simulink model "AeroModel"  (R2024b)
settings: Solver=VariableStepAuto  StartTime=0.0  StopTime=10.0  RelTol=1e-3
settings Model: Creator=ewise  LastModifiedBy=ewise

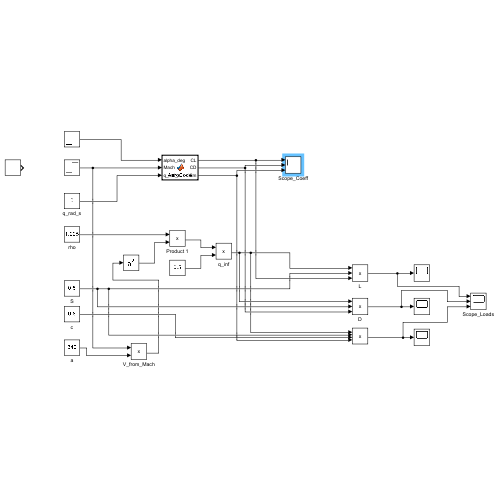
[thumbnail: Simulink's stored preview of the top-level diagram]
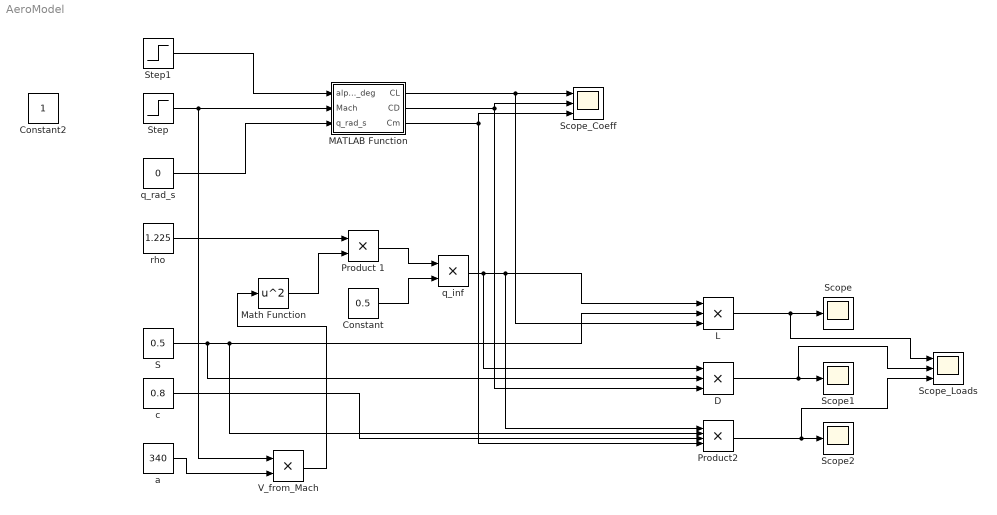
== system AeroModel ==
  Constant : Constant  Value=0.5
  Constant2 : Constant
  D : Product  Inputs=3
  L : Product  Inputs=3
  MATLAB Function : MATLAB Function  TreatAsAtomicUnit=on
  Math Function : Math  Operator=square
  Product 1 : Product
  Product2 : Product  Inputs=4
  S : Constant  Value=0.5
  Scope : Scope
  Scope1 : Scope
  Scope2 : Scope
  Scope_Coeff : Scope  NumInputPorts=3
  Scope_Loads : Scope  NumInputPorts=3
  Step : Step  Time=3  Before=4  After=7  SampleTime=0
  Step1 : Step  Time=2  Before=2  After=12  SampleTime=0
  V_from_Mach : Product
  a : Constant  Value=340
  c : Constant  Value=0.8
  q_inf : Product
  q_rad_s : Constant  Value=0
  rho : Constant  Value=1.225
  wires:
  Step/1 -> V_from_Mach/1, MATLAB Function/2(Mach)
  q_rad_s/1 -> MATLAB Function/3(q_rad_s)
  MATLAB Function/2(CD) -> Scope_Coeff/2, D/3
  MATLAB Function/3(Cm) -> Product2/4, Scope_Coeff/3
  rho/1 -> Product 1/1
  Math Function/1 -> Product 1/2
  Product 1/1 -> q_inf/1
  Constant/1 -> q_inf/2
  q_inf/1 -> D/1, Product2/1, L/1
  S/1 -> D/2, Product2/2, L/2
  MATLAB Function/1(CL) -> Scope_Coeff/1, L/3
  c/1 -> Product2/3
  L/1 -> Scope_Loads/1, Scope/1
  D/1 -> Scope_Loads/2, Scope1/1
  Product2/1 -> Scope_Loads/3, Scope2/1
  a/1 -> V_from_Mach/2
  V_from_Mach/1 -> Math Function/1
  Step1/1 -> MATLAB Function/1(alpha_deg)

== matlab function AeroModel/MATLAB Function ==
  data: alpha_deg input; CL output; Mach input; q_rad_s input; CD output; Cm output
function [CL, CD, Cm] = AeroCode(alpha_deg, Mach, q_rad_s)
%#codegen
% Simulink-safe polynomial surrogate (no workspace access)

% ---- Paste your trained constants here ----
muX = [7.4735,    5.5013,   -0.0009];      % aeroModel.muX from MATLAB script
sgX = [7.3342,    1.4811,    1.2011];      % <-- replace with aeroModel.sgX (no zeros)
W = [ ...
    0.6674,  0.2166, -0.1027;
    0.7657,  0.2806, -0.1137;
    0.0512,  0.0229, -0.0053;
    0.0000,  0.0000, -0.0775;
   -0.0140,  0.1468,  0.0011;
   -0.0000, -0.0000,  0.0000;
   -0.0001,  0.0000,  0.0000;
    0.0471,  0.0081, -0.0052;
    0.0001, -0.0000, -0.0000;
    0.0002, -0.0000, -0.0032];      % <-- replace with aeroModel.W (10x3)

% Normalize inputs
aN = (alpha_deg - muX(1)) / sgX(1);
mN = (Mach      - muX(2)) / sgX(2);
qN = (q_rad_s   - muX(3)) / sgX(3);

% Feature vector: [1 a m q a^2 m^2 q^2 a*m a*q m*q]
Phi = [1, aN, mN, qN, aN*aN, mN*mN, qN*qN, aN*mN, aN*qN, mN*qN];

% Predict [CL CD Cm]
C = Phi * W;

CL = C(1);
CD = C(2);
Cm = C(3);
end
